simulink model "TD3_Ex_sim_part3"  (R2022a)
settings: Solver=VariableStepAuto  StartTime=0.0  StopTime=10.0  RelTol=1e-3
undefined symbols (not defined in the file): A, A_obs, A_obs_Kal, B, B_obs, B_obs_Kal, C, C_obs, D_obs, K_LQ, l_LQ, xinit_obs
libraries: simulink x2
settings Model: Creator=CS  LastModifiedBy=CS

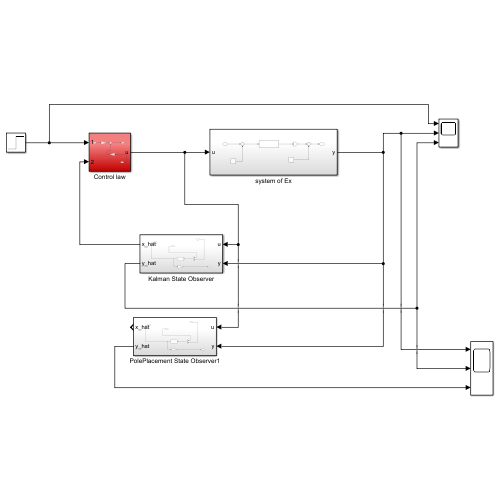
[thumbnail: Simulink's stored preview of the top-level diagram]
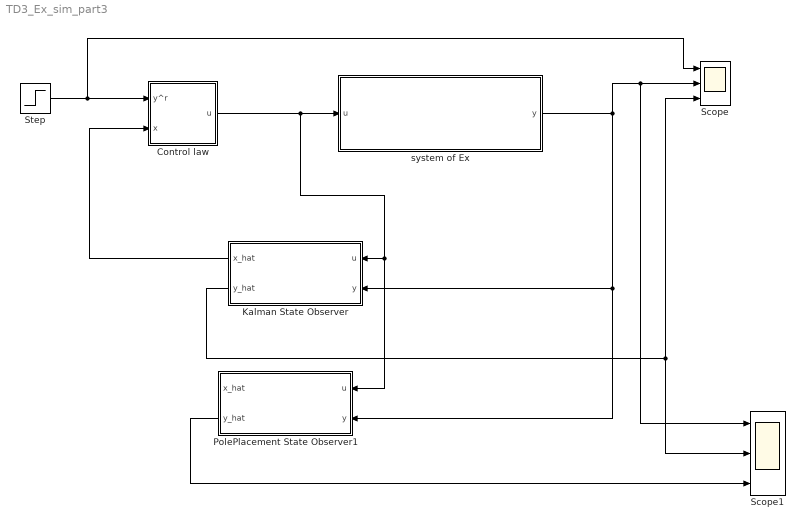
== system TD3_Ex_sim_part3 ==
  Control law : Subsystem
  Kalman State Observer : Subsystem
  PolePlacement State Observer1 : Subsystem
  Scope : Scope  NumInputPorts=3
  Scope1 : Scope  NumInputPorts=3
  Step : Step  SampleTime=0
  system of Ex : Subsystem
  wires:
  Step/1 -> Control law/1(y^r), Scope/1
  system of Ex/1(y) -> Scope1/1, Scope/2, PolePlacement State Observer1/2(y), Kalman State Observer/2(y)
  Control law/1(u) -> system of Ex/1(u), PolePlacement State Observer1/1(u), Kalman State Observer/1(u)
  Kalman State Observer/2(y_hat) -> Scope1/2, Scope/3
  Kalman State Observer/1(x_hat) -> Control law/2(x)
  PolePlacement State Observer1/2(y_hat) -> Scope1/3

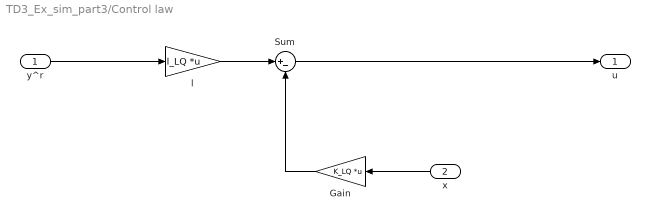
== system TD3_Ex_sim_part3/Control law ==
  y^r : Inport
  x : Inport  Port=2
  Gain : Gain  Gain=K_LQ  Multiplication=Matrix(K*u) (u vector)
  Sum : Sum  Inputs=|+-
  l : Gain  Gain=l_LQ  Multiplication=Matrix(K*u) (u vector)
  u : Outport
  wires:
  Gain/1 -> Sum/2
  Sum/1 -> u/1
  l/1 -> Sum/1
  x/1 -> Gain/1
  y^r/1 -> l/1

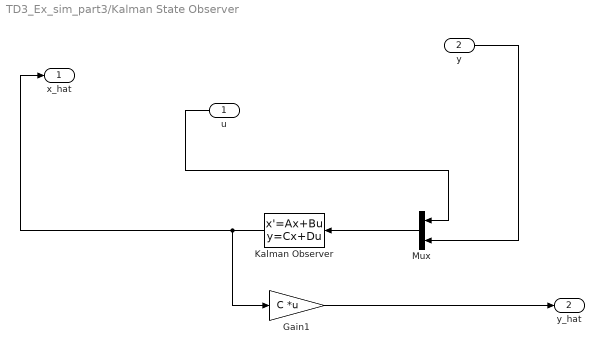
== system TD3_Ex_sim_part3/Kalman State Observer ==
  u : Inport
  y : Inport  Port=2
  Gain1 : Gain  Gain=C  Multiplication=Matrix(K*u) (u vector)
  Kalman Observer : StateSpace  A=A_obs_Kal  B=B_obs_Kal  C=C_obs  D=D_obs  InitialCondition=xinit_obs
  Mux : Mux  Inputs=2
  x_hat : Outport
  y_hat : Outport  Port=2
  wires:
  Kalman Observer/1 -> x_hat/1, Gain1/1
  Gain1/1 -> y_hat/1
  y/1 -> Mux/2
  Mux/1 -> Kalman Observer/1
  u/1 -> Mux/1

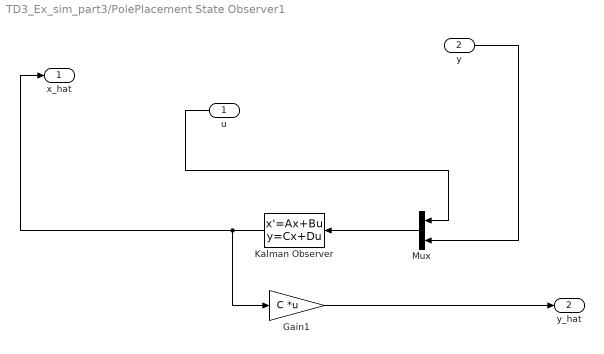
== system TD3_Ex_sim_part3/PolePlacement State Observer1 ==
  u : Inport
  y : Inport  Port=2
  Gain1 : Gain  Gain=C  Multiplication=Matrix(K*u) (u vector)
  Kalman Observer : StateSpace  A=A_obs  B=B_obs  C=C_obs  D=D_obs  InitialCondition=xinit_obs
  Mux : Mux  Inputs=2
  x_hat : Outport
  y_hat : Outport  Port=2
  wires:
  Kalman Observer/1 -> x_hat/1, Gain1/1
  Gain1/1 -> y_hat/1
  y/1 -> Mux/2
  Mux/1 -> Kalman Observer/1
  u/1 -> Mux/1

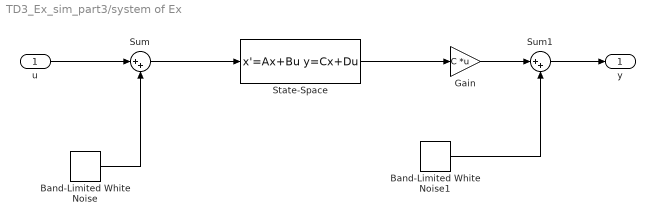
== system TD3_Ex_sim_part3/system of Ex ==
  u : Inport
  Band-Limited White Noise : simulink/Sources/Band-Limited White Noise  Cov=du0  Ts=0.01  seed=[23341]
  Band-Limited White Noise1 : simulink/Sources/Band-Limited White Noise  Cov=dy0  Ts=0.01  seed=[23341]
  Gain : Gain  Gain=C  Multiplication=Matrix(K*u) (u vector)
  State-Space : StateSpace  A=A  B=B  C=eye(3)  D=zeros(3,1)  InitialCondition=0
  Sum : Sum  Inputs=|++
  Sum1 : Sum  Inputs=|++
  y : Outport
  wires:
  State-Space/1 -> Gain/1
  u/1 -> Sum/1
  Sum/1 -> State-Space/1
  Gain/1 -> Sum1/1
  Sum1/1 -> y/1
  Band-Limited White Noise/1 -> Sum/2
  Band-Limited White Noise1/1 -> Sum1/2
